simulink model "stereo_ibvs_core_backup_20260724_173834"  (R2025b)
settings: Solver=FixedStepDiscrete  StartTime=0.0  StopTime=10  FixedStep=cfg.Ts  RelTol=1e-3
InitFcn:
  | modelPath = get_param(bdroot,'FileName');
  |                                                                                       simulinkPath = fileparts(fileparts(modelPath));
  |                                                                                       configPath = fullfile(simulinkPath,'config','stereo_ibvs_config.m');
  |                                                                                       if ~isfile(configPath), error('StereoIBVS:ConfigNotFound','找不到配置文件：%s',configPath); end
  |                                                                                       run(configPath);
undefined symbols (not defined in the file): cfg
(part 3 of 4)

== matlab function stereo_ibvs_core_backup_20260724_173834/04_FR3_Camera_Kinematics/FR3 Camera Kinematics ==
  data: q input; pWCL output; cfg_T_W_B input; cfg_fr3OriginXYZ input; cfg_fr3OriginRPY input; cfg_fr3Axis input; cfg_fr3Joint8OriginXYZ input; cfg_fr3Joint8OriginRPY input; cfg_T_link8_CL input; cfg_T_CL_CR input; cfg_numericalEpsilon input; RWCL output; pWCR output; RWCR output; JL output; JR output; rankJL output; rcondJL output; rotationOrthogonalityError output; baselineLength output; baselineError output; stereoRotationError output; pWLink8 output; RWLink8 output; kinematicsValid output
function [ ...
    pWCL, ...
    RWCL, ...
    pWCR, ...
    RWCR, ...
    JL, ...
    JR, ...
    rankJL, ...
    rcondJL, ...
    rotationOrthogonalityError, ...
    baselineLength, ...
    baselineError, ...
    stereoRotationError, ...
    pWLink8, ...
    RWLink8, ...
    kinematicsValid] = fcn( ...
    q, ...
    cfg_T_W_B, ...
    cfg_fr3OriginXYZ, ...
    cfg_fr3OriginRPY, ...
    cfg_fr3Axis, ...
    cfg_fr3Joint8OriginXYZ, ...
    cfg_fr3Joint8OriginRPY, ...
    cfg_T_link8_CL, ...
    cfg_T_CL_CR, ...
    cfg_numericalEpsilon)
%#codegen
% V2 FR3双目相机运动学与诊断。

% 固定尺寸输出
pWCL = zeros(3,1);
RWCL = eye(3);
pWCR = zeros(3,1);
RWCR = eye(3);
JL = zeros(6,7);
JR = zeros(6,7);
rankJL = 0;
rcondJL = 0;
rotationOrthogonalityError = 0;
baselineLength = 0;
baselineError = 0;
stereoRotationError = 0;
pWLink8 = zeros(3,1);
RWLink8 = eye(3);
kinematicsValid = false;

% 输入整理和检查
qSafe = reshape(q,7,1);

inputValid = ...
    all(isfinite(qSafe)) && ...
    all(isfinite(cfg_T_W_B(:))) && ...
    all(isfinite(cfg_fr3OriginXYZ(:))) && ...
    all(isfinite(cfg_fr3OriginRPY(:))) && ...
    all(isfinite(cfg_fr3Axis(:))) && ...
    all(isfinite(cfg_fr3Joint8OriginXYZ(:))) && ...
    all(isfinite(cfg_fr3Joint8OriginRPY(:))) && ...
    all(isfinite(cfg_T_link8_CL(:))) && ...
    all(isfinite(cfg_T_CL_CR(:))) && ...
    isfinite(cfg_numericalEpsilon) && ...
    cfg_numericalEpsilon > 0;

if ~inputValid
    return;
end

% FR3正运动学
T = reshape(cfg_T_W_B,4,4);
jointOriginsW = zeros(3,7);
jointAxesW = zeros(3,7);

for jointIndex = 1:7
    T = T * makeTransform( ...
        cfg_fr3OriginXYZ(:,jointIndex), ...
        cfg_fr3OriginRPY(:,jointIndex));

    jointOriginsW(:,jointIndex) = T(1:3,4);

    axisLocal = cfg_fr3Axis(:,jointIndex);
    axisNorm = norm(axisLocal);

    if ~isfinite(axisNorm) || ...
            axisNorm <= cfg_numericalEpsilon
        return;
    end

    jointAxesW(:,jointIndex) = ...
        T(1:3,1:3) * axisLocal;

    T = T * axisRotation(axisLocal,qSafe(jointIndex));
end

% link8固定变换
T_W_link8 = T * makeTransform( ...
    cfg_fr3Joint8OriginXYZ, ...
    cfg_fr3Joint8OriginRPY);

pWLink8 = T_W_link8(1:3,4);
RWLink8 = T_W_link8(1:3,1:3);

% 左右相机位姿
T_W_CL = T_W_link8 * reshape(cfg_T_link8_CL,4,4);
T_W_CR = T_W_CL * reshape(cfg_T_CL_CR,4,4);

pWCL = T_W_CL(1:3,4);
RWCL = T_W_CL(1:3,1:3);
pWCR = T_W_CR(1:3,4);
RWCR = T_W_CR(1:3,1:3);

% 左相机光心的世界坐标Jacobian
JWLeft = zeros(6,7);

for jointIndex = 1:7
    JWLeft(1:3,jointIndex) = cross( ...
        jointAxesW(:,jointIndex), ...
        pWCL-jointOriginsW(:,jointIndex));

    JWLeft(4:6,jointIndex) = ...
        jointAxesW(:,jointIndex);
end

% 转换到左相机坐标系
R_CL_W = RWCL';

JL = [ ...
    R_CL_W, zeros(3,3)
    zeros(3,3), R_CL_W
    ] * JWLeft;

% 从左相机Jacobian转换到右相机坐标系
R_CL_CR = cfg_T_CL_CR(1:3,1:3);
p_CL_CR = cfg_T_CL_CR(1:3,4);

JR = [ ...
    R_CL_CR', -R_CL_CR'*skew3(p_CL_CR)
    zeros(3,3), R_CL_CR'
    ] * JL;

% 有限值检查
finiteResult = ...
    all(isfinite(pWCL)) && ...
    all(isfinite(RWCL(:))) && ...
    all(isfinite(pWCR)) && ...
    all(isfinite(RWCR(:))) && ...
    all(isfinite(JL(:))) && ...
    all(isfinite(JR(:))) && ...
    all(isfinite(pWLink8)) && ...
    all(isfinite(RWLink8(:)));

if ~finiteResult
    pWCL = zeros(3,1);
    RWCL = eye(3);
    pWCR = zeros(3,1);
    RWCR = eye(3);
    JL = zeros(6,7);
    JR = zeros(6,7);
    pWLink8 = zeros(3,1);
    RWLink8 = eye(3);
    return;
end

% V2运动学诊断
rankJL = rank(JL);
rcondJL = rcond(JL*JL');

rotationOrthogonalityError = max([ ...
    norm(RWCL'*RWCL-eye(3),'fro'), ...
    norm(RWCR'*RWCR-eye(3),'fro'), ...
    norm(RWLink8'*RWLink8-eye(3),'fro')]);

baselineLength = norm(pWCR-pWCL);
baselineError = abs( ...
    baselineLength-norm(p_CL_CR));

stereoRotationError = norm( ...
    RWCR-RWCL*R_CL_CR, ...
    'fro');

% 最终有效性判断
rotationTolerance = max( ...
    1e-6, ...
    100*cfg_numericalEpsilon);

diagnosticsFinite = ...
    isfinite(rankJL) && ...
    isfinite(rcondJL) && ...
    isfinite(rotationOrthogonalityError) && ...
    isfinite(baselineLength) && ...
    isfinite(baselineError) && ...
    isfinite(stereoRotationError);

rotationValid = ...
    rotationOrthogonalityError <= rotationTolerance && ...
    abs(det(RWCL)-1) <= rotationTolerance && ...
    abs(det(RWCR)-1) <= rotationTolerance && ...
    abs(det(RWLink8)-1) <= rotationTolerance;

kinematicsValid = ...
    diagnosticsFinite && ...
    rotationValid;

if ~kinematicsValid
    return;
end
end


function T = makeTransform(xyz,rpy)
T = eye(4);
T(1:3,1:3) = ...
    rotz3(rpy(3)) * ...
    roty3(rpy(2)) * ...
    rotx3(rpy(1));
T(1:3,4) = xyz;
end


function T = axisRotation(axis,q)
axisNorm = norm(axis);
unitAxis = axis / axisNorm;
K = skew3(unitAxis);
R = eye(3) + ...
    sin(q)*K + ...
    (1-cos(q))*(K*K);
T = eye(4);
T(1:3,1:3) = R;
end


function R = rotx3(angle)
c = cos(angle);
s = sin(angle);
R = [ ...
    1, 0, 0
    0, c, -s
    0, s, c
    ];
end


function R = roty3(angle)
c = cos(angle);
s = sin(angle);
R = [ ...
    c, 0, s
    0, 1, 0
    -s, 0, c
    ];
end


function R = rotz3(angle)
c = cos(angle);
s = sin(angle);
R = [ ...
    c, -s, 0
    s, c, 0
    0, 0, 1
    ];
end


function S = skew3(vector)
S = [ ...
    0, -vector(3), vector(2)
    vector(3), 0, -vector(1)
    -vector(2), vector(1), 0
    ];
end

== matlab function stereo_ibvs_core_backup_20260724_173834/05_Target_EKF/V2 Target EKF ==
  data: zMeasured input; pHatW output; measurementEnable input; visionMeasurementNewSafe input; pWCL input; RWCL input; fxMeasuredPx input; fyMeasuredPx input; resetSafe input; cfg_ekfX0 input; cfg_ekfP0 input; cfg_Ts input; cfg_sigmaJerk input; cfg_visibilityZMin input; cfg_numericalEpsilon input; cfg_rhoMin input; cfg_rhoMax input; cfg_pixelNoiseStd input; cfg_baseline input; cfg_ekfCovarianceJitter input; cfg_ekfSConditionMin input; cfg_ekfInitializationMode input; cfg_ekfRequireNewMeasurement input; vHatW output; aHatW output; pHatLeft output; vHatLeft output; rhoHatRaw output; rhoHatSafe output; innovation output; rhoInnovation output; innovationNorm output; traceP output; ekfPredictionValid output; ekfMeasurementUpdated output; ekfStateFinite output; minEigenvalueP output; symmetryErrorP output
function [ ...
    pHatW, ...
    vHatW, ...
    aHatW, ...
    pHatLeft, ...
    vHatLeft, ...
    rhoHatRaw, ...
    rhoHatSafe, ...
    innovation, ...
    rhoInnovation, ...
    innovationNorm, ...
    traceP, ...
    ekfPredictionValid, ...
    ekfMeasurementUpdated, ...
    ekfStateFinite, ...
    minEigenvalueP, ...
    symmetryErrorP] = fcn( ...
    zMeasured, ...
    measurementEnable, ...
    visionMeasurementNewSafe, ...
    pWCL, ...
    RWCL, ...
    fxMeasuredPx, ...
    fyMeasuredPx, ...
    resetSafe, ...
    cfg_ekfX0, ...
    cfg_ekfP0, ...
    cfg_Ts, ...
    cfg_sigmaJerk, ...
    cfg_visibilityZMin, ...
    cfg_numericalEpsilon, ...
    cfg_rhoMin, ...
    cfg_rhoMax, ...
    cfg_pixelNoiseStd, ...
    cfg_baseline, ...
    cfg_ekfCovarianceJitter, ...
    cfg_ekfSConditionMin, ...
    cfg_ekfInitializationMode, ...
    cfg_ekfRequireNewMeasurement)
%#codegen
% V2九状态世界坐标恒加速度EKF。
% 首次有效双目测量可直接初始化目标世界坐标位置。

% 固定尺寸输出
pHatW = zeros(3,1);
vHatW = zeros(3,1);
aHatW = zeros(3,1);
pHatLeft = zeros(3,1);
vHatLeft = zeros(3,1);
rhoHatRaw = 0;
rhoHatSafe = 0;
innovation = zeros(3,1);
rhoInnovation = 0;
innovationNorm = 0;
traceP = 0;
ekfPredictionValid = 0;
ekfMeasurementUpdated = 0;
ekfStateFinite = 0;
minEigenvalueP = 0;
symmetryErrorP = 0;

% 输入整理
z = reshape(zMeasured,3,1);
pCameraW = reshape(pWCL,3,1);
rotationCameraToWorld = reshape(RWCL,3,3);
fx = reshape(fxMeasuredPx,2,1);
fy = reshape(fyMeasuredPx,2,1);
ekfX0 = reshape(cfg_ekfX0,9,1);
ekfP0 = reshape(cfg_ekfP0,9,9);

% 持久状态
persistent x P initialized

if isempty(x)
    x = zeros(9,1);
    P = eye(9);
    initialized = false;
end

% 配置和输入有效性
configurationValid = ...
    all(isfinite(ekfX0)) && ...
    all(isfinite(ekfP0(:))) && ...
    isfinite(cfg_Ts) && cfg_Ts > 0 && ...
    isfinite(cfg_sigmaJerk) && cfg_sigmaJerk >= 0 && ...
    isfinite(cfg_visibilityZMin) && cfg_visibilityZMin > 0 && ...
    isfinite(cfg_numericalEpsilon) && cfg_numericalEpsilon > 0 && ...
    isfinite(cfg_rhoMin) && ...
    isfinite(cfg_rhoMax) && ...
    cfg_rhoMax > cfg_rhoMin && ...
    isfinite(cfg_pixelNoiseStd) && cfg_pixelNoiseStd >= 0 && ...
    isfinite(cfg_baseline) && ...
    cfg_baseline > cfg_numericalEpsilon && ...
    isfinite(cfg_ekfCovarianceJitter) && ...
    cfg_ekfCovarianceJitter >= 0 && ...
    isfinite(cfg_ekfSConditionMin) && ...
    cfg_ekfSConditionMin >= 0 && ...
    isfinite(cfg_ekfInitializationMode) && ...
    isfinite(cfg_ekfRequireNewMeasurement);

kinematicInputFinite = ...
    all(isfinite(pCameraW)) && ...
    all(isfinite(rotationCameraToWorld(:)));

focalPixelsValid = ...
    all(isfinite(fx)) && ...
    all(isfinite(fy)) && ...
    all(fx > cfg_numericalEpsilon) && ...
    all(fy > cfg_numericalEpsilon);

measurementEnableValid = ...
    isfinite(measurementEnable) && ...
    measurementEnable > 0.5;

visionNewValid = ...
    isfinite(visionMeasurementNewSafe) && ...
    visionMeasurementNewSafe > 0.5;

newMeasurementAccepted = ...
    cfg_ekfRequireNewMeasurement <= 0.5 || ...
    visionNewValid;

measurementFinite = all(isfinite(z));
measurementRhoValid = ...
    measurementFinite && ...
    z(3) >= cfg_rhoMin && ...
    z(3) <= cfg_rhoMax;

measurementAvailable = ...
    configurationValid && ...
    measurementEnableValid && ...
    newMeasurementAccepted && ...
    kinematicInputFinite && ...
    focalPixelsValid && ...
    measurementRhoValid;

resetRequested = ...
    isfinite(resetSafe) && ...
    resetSafe > 0.5;

if ~configurationValid
    initialized = false;
    return;
end

if resetRequested
    x = ekfX0;
    P = ekfP0;
    initialized = false;
    return;
end

% 固定初值模式兼容
fixedInitializationMode = ...
    cfg_ekfInitializationMode <= 0.5;

if ~initialized && fixedInitializationMode
    x = ekfX0;
    P = ekfP0;
    initialized = true;
end

% 首次有效双目测量初始化
justInitialized = false;

if ~initialized && measurementAvailable
    rhoInitial = z(3);
    depthInitial = 1/rhoInitial;

    pInitialLeft = [ ...
        z(1)*depthInitial
        z(2)*depthInitial
        depthInitial
    ];

    pInitialW = ...
        pCameraW + ...
        rotationCameraToWorld*pInitialLeft;

    initializationFinite = ...
        all(isfinite(pInitialLeft)) && ...
        all(isfinite(pInitialW)) && ...
        depthInitial > cfg_visibilityZMin;

    if initializationFinite
        x = [ ...
            pInitialW
            zeros(3,1)
            zeros(3,1)
        ];
        P = ekfP0;
        initialized = true;
        justInitialized = true;
        ekfMeasurementUpdated = 1;
    end
end

% 尚未初始化时保持安全无效输出
if ~initialized
    traceP = trace(0.5*(P+P'));
    return;
end

% 初始化当周期不重复执行预测和测量更新
if justInitialized
    pHatW = x(1:3);
    vHatW = x(4:6);
    aHatW = x(7:9);
    pHatLeft = ...
        rotationCameraToWorld' * ...
        (pHatW-pCameraW);
    vHatLeft = rotationCameraToWorld'*vHatW;

    ekfStateFinite = double( ...
        all(isfinite(x)) && ...
        all(isfinite(P(:))) && ...
        all(isfinite(pHatLeft)) && ...
        all(isfinite(vHatLeft)));

    if ekfStateFinite > 0.5 && ...
            pHatLeft(3) > cfg_visibilityZMin
        rhoHatRaw = 1/pHatLeft(3);
        rhoHatSafe = min( ...
            max(rhoHatRaw,cfg_rhoMin), ...
            cfg_rhoMax);
        ekfPredictionValid = 1;
    end

    Psym = 0.5*(P+P');
    traceP = trace(Psym);
    symmetryErrorP = norm(P-P','fro');
    eigenvaluesP = eig(Psym);
    minEigenvalueP = min(real(eigenvaluesP));
    return;
end

% 恒加速度状态模型
I3 = eye(3);
Z3 = zeros(3,3);
I9 = eye(9);
Ts = cfg_Ts;

F = [ ...
    I3, Ts*I3, 0.5*Ts*Ts*I3
    Z3, I3,    Ts*I3
    Z3, Z3,    I3
];

sigmaJerkSquared = cfg_sigmaJerk*cfg_sigmaJerk;

Q = sigmaJerkSquared * [ ...
    (Ts^5/20)*I3, (Ts^4/8)*I3, (Ts^3/6)*I3
    (Ts^4/8)*I3,  (Ts^3/3)*I3, (Ts^2/2)*I3
    (Ts^3/6)*I3,  (Ts^2/2)*I3, Ts*I3
];

% 预测
xPred = F*x;
PPred = F*P*F' + Q;
PPred = 0.5*(PPred+PPred');

pPredW = xPred(1:3);
pPredLeft = ...
    rotationCameraToWorld' * ...
    (pPredW-pCameraW);

predictionFinite = ...
    kinematicInputFinite && ...
    all(isfinite(xPred)) && ...
    all(isfinite(PPred(:))) && ...
    all(isfinite(pPredLeft));

ekfPredictionValid = double( ...
    predictionFinite && ...
    pPredLeft(3) > cfg_visibilityZMin);

% 默认采用预测结果
x = xPred;
P = PPred;

% 仅在新视觉消息到来时执行测量更新
measurementOK = ...
    measurementAvailable && ...
    ekfPredictionValid > 0.5;

if measurementOK
    Z = pPredLeft(3);
    rhoPred = 1/Z;
    xLeftPred = pPredLeft(1)/Z;
    yLeftPred = pPredLeft(2)/Z;

    h = [xLeftPred; yLeftPred; rhoPred];

    HLeft = [ ...
        rhoPred, 0,       -xLeftPred*rhoPred
        0,       rhoPred, -yLeftPred*rhoPred
        0,       0,       -rhoPred*rhoPred
    ];

    HWorld = HLeft*rotationCameraToWorld';
    H = [HWorld, zeros(3,3), zeros(3,3)];

    if all(isfinite(h)) && all(isfinite(H(:)))
        innovation = z-h;
        rhoInnovation = innovation(3);

        pixelVariance = ...
            cfg_pixelNoiseStd*cfg_pixelNoiseStd;
        fxLeft = max(fx(1),cfg_numericalEpsilon);
        fxRight = max(fx(2),cfg_numericalEpsilon);
        fyLeft = max(fy(1),cfg_numericalEpsilon);
        baseline = max(cfg_baseline,cfg_numericalEpsilon);

        varXLeft = pixelVariance/(fxLeft*fxLeft);
        varYLeft = pixelVariance/(fyLeft*fyLeft);
        covXLeftRho = ...
            pixelVariance/(baseline*fxLeft*fxLeft);
        varRho = pixelVariance/(baseline*baseline) * ...
            (1/(fxLeft*fxLeft)+1/(fxRight*fxRight));

        R = [ ...
            varXLeft,    0,        covXLeftRho
            0,           varYLeft, 0
            covXLeftRho, 0,        varRho
        ];

        R = R + cfg_ekfCovarianceJitter*eye(3);
        S = H*PPred*H' + R;

        innovationCovarianceValid = ...
            all(isfinite(S(:))) && ...
            rcond(S) > cfg_ekfSConditionMin;

        if innovationCovarianceValid
            K = (PPred*H')/S;
            xUpdated = xPred+K*innovation;
            A = I9-K*H;
            PUpdated = A*PPred*A'+K*R*K';
            PUpdated = 0.5*(PUpdated+PUpdated');

            if cfg_ekfCovarianceJitter > 0
                PUpdated = PUpdated + ...
                    cfg_ekfCovarianceJitter*I9;
            end

            updateFinite = ...
                all(isfinite(xUpdated)) && ...
                all(isfinite(PUpdated(:)));

            if updateFinite
                x = xUpdated;
                P = PUpdated;
                ekfMeasurementUpdated = 1;
            end
        end
    end
end

% 状态输出
pHatW = x(1:3);
vHatW = x(4:6);
aHatW = x(7:9);
pHatLeft = ...
    rotationCameraToWorld' * ...
    (pHatW-pCameraW);
vHatLeft = rotationCameraToWorld'*vHatW;

ekfStateFinite = double( ...
    all(isfinite(x)) && ...
    all(isfinite(P(:))) && ...
    all(isfinite(pHatLeft)) && ...
    all(isfinite(vHatLeft)));

if ekfStateFinite > 0.5 && ...
        pHatLeft(3) > cfg_visibilityZMin
    rhoHatRaw = 1/pHatLeft(3);
    rhoHatSafe = min( ...
        max(rhoHatRaw,cfg_rhoMin), ...
        cfg_rhoMax);
else
    rhoHatRaw = 0;
    rhoHatSafe = 0;
    ekfPredictionValid = 0;
end

innovationNorm = sqrt(innovation'*innovation);
Psym = 0.5*(P+P');
symmetryErrorP = norm(P-P','fro');
traceP = trace(Psym);
eigenvaluesP = eig(Psym);
minEigenvalueP = min(real(eigenvaluesP));

% 非有限状态自动复位并重新等待初始化
diagnosticsValid = ...
    ekfStateFinite > 0.5 && ...
    isfinite(traceP) && ...
    isfinite(minEigenvalueP) && ...
    isfinite(symmetryErrorP);

if ~diagnosticsValid
    x = ekfX0;
    P = ekfP0;
    initialized = false;

    pHatW = zeros(3,1);
    vHatW = zeros(3,1);
    aHatW = zeros(3,1);
    pHatLeft = zeros(3,1);
    vHatLeft = zeros(3,1);
    rhoHatRaw = 0;
    rhoHatSafe = 0;
    innovation = zeros(3,1);
    rhoInnovation = 0;
    innovationNorm = 0;
    traceP = trace(ekfP0);
    minEigenvalueP = 0;
    symmetryErrorP = 0;
    ekfPredictionValid = 0;
    ekfMeasurementUpdated = 0;
    ekfStateFinite = 0;
end
end

== matlab function stereo_ibvs_core_backup_20260724_173834/06_Estimated_Rho_Dynamics/Estimate Rho Dynamics ==
  data: normalizedFeatureMeasured input; rhoDotHat output; rhoHatSafe input; vHatCL input; vHatCR input; JL input; JR input; qDotMeasured input; motionFeedbackValid input; cfg_numericalEpsilon input; rhoDynamicsValid output
function [rhoDotHat, rhoDynamicsValid] = fcn( ...
    normalizedFeatureMeasured, ...
    rhoHatSafe, ...
    vHatCL, ...
    vHatCR, ...
    JL, ...
    JR, ...
    qDotMeasured, ...
    motionFeedbackValid, ...
    cfg_numericalEpsilon)
%#codegen
% 本函数使用实测关节速度估计左右相机运动引起的逆深度变化率。
%
% 输入尺寸：
% normalizedFeatureMeasured : 4×1 [xL;yL;xR;yR]
% rhoHatSafe                : 1×1
% vHatCL                    : 3×1
% vHatCR                    : 3×1
% JL                        : 6×7
% JR                        : 6×7
% qDotMeasured              : 7×1，来自JointState.velocity
% motionFeedbackValid       : 1×1
%
% 输出：
% rhoDotHat                 : 2×1
% rhoDynamicsValid          : 1×1

%% 固定尺寸输出
rhoDotHat = zeros(2,1);
rhoDynamicsValid = false;

features = reshape(normalizedFeatureMeasured,4,1);
velocityCL = reshape(vHatCL,3,1);
velocityCR = reshape(vHatCR,3,1);
qDotFeedback = reshape(qDotMeasured,7,1);

%% 输入有效性
inputValid = ...
    all(isfinite(features)) && ...
    isfinite(rhoHatSafe) && ...
    all(isfinite(velocityCL)) && ...
    all(isfinite(velocityCR)) && ...
    all(isfinite(JL(:))) && ...
    all(isfinite(JR(:))) && ...
    all(isfinite(qDotFeedback)) && ...
    isfinite(motionFeedbackValid) && ...
    motionFeedbackValid > 0.5 && ...
    isfinite(cfg_numericalEpsilon) && ...
    cfg_numericalEpsilon > 0 && ...
    rhoHatSafe > cfg_numericalEpsilon;

if ~inputValid
    return;
end

rho = max(rhoHatSafe, cfg_numericalEpsilon);

%% 左相机
xL = features(1);
yL = features(2);

LrhoL = [
    0, 0, rho*rho, ...
    rho*yL, -rho*xL, 0
];

Hrho = [0, 0, -rho*rho];

cameraVelocityLeft = JL * qDotFeedback;

rhoDotHat(1) = ...
    LrhoL * cameraVelocityLeft + ...
    Hrho * velocityCL;

%% 右相机
xR = features(3);
yR = features(4);

LrhoR = [
    0, 0, rho*rho, ...
    rho*yR, -rho*xR, 0
];

cameraVelocityRight = JR * qDotFeedback;

rhoDotHat(2) = ...
    LrhoR * cameraVelocityRight + ...
    Hrho * velocityCR;

%% 最终数值保护
if all(isfinite(rhoDotHat))
    rhoDynamicsValid = true;
else
    rhoDotHat = zeros(2,1);
    rhoDynamicsValid = false;
end
end

== matlab function stereo_ibvs_core_backup_20260724_173834/07_Arm_Priority_Controller/Final Arm Priority Controller ==
  data: q input; qDotCmd output; cLMeasured input; rhoHatL input; vHatLeft input; JL input; cLd input; rhoD input; validLeft input; ekfPredictionValid input; centerEnable input; depthEnable input; armEnable input; depthTaskWeight input; cfg_numericalEpsilon input; cfg_robustEnable input; cfg_betaC input; cfg_epsilonC input; cfg_Kc input; cfg_lambdaC input; cfg_betaRho input; cfg_epsilonRho input; cfg_kRho input; cfg_lambdaRho input; cfg_nullspaceEnable input; cfg_kNull input; cfg_qMid input; cfg_leftOnlyCenterControlEnable input; centerError output; depthError output; rcondJc output; rcondArho output; qDotCenter output; qDotDepthRaw output; qDotDepthWeighted output; qDotNullUsed output
function [qDotCmd,centerError,depthError,rcondJc,rcondArho,qDotCenter,qDotDepthRaw,qDotDepthWeighted,qDotNullUsed] = ...
    fcn(q,cLMeasured,rhoHatL,vHatLeft,JL,cLd,rhoD,validLeft,ekfPredictionValid,centerEnable,depthEnable,armEnable,depthTaskWeight, ...
    cfg_numericalEpsilon,cfg_robustEnable,cfg_betaC,cfg_epsilonC,cfg_Kc,cfg_lambdaC,cfg_betaRho,cfg_epsilonRho,cfg_kRho,cfg_lambdaRho,cfg_nullspaceEnable,cfg_kNull,cfg_qMid,cfg_leftOnlyCenterControlEnable)
%#codegen
% 代码作用：
% 左相机归一化中心为主任务，逆深度为次任务。
% 支持目标速度前馈、鲁棒项、阻尼伪逆和关节中位零空间任务。

qDotCmd = zeros(7,1);
centerError = zeros(2,1);
depthError = 0;
rcondJc = 0;
rcondArho = 0;
qDotCenter = zeros(7,1);
qDotDepthRaw = zeros(7,1);
qDotDepthWeighted = zeros(7,1);
qDotNullUsed = zeros(7,1);

x = cLMeasured(1);
y = cLMeasured(2);
rho = rhoD;
vFeed = zeros(3,1);

if ekfPredictionValid > 0.5 && ...
        isfinite(rhoHatL) && rhoHatL > 0 && ...
        all(isfinite(vHatLeft))
    rho = max(rhoHatL,cfg_numericalEpsilon);
    vFeed = vHatLeft;
end

centerError = [x;y] - cLd;
depthError = rho - rhoD;

Lc = [
    -rho, 0, x*rho, x*y, -(1+x*x), y
    0, -rho, y*rho, 1+y*y, -x*y, -x
];

Hc = rho*[1 0 -x;0 1 -y];
bhatC = Hc*vFeed;
Jc = Lc*JL;

rc = zeros(2,1);
if cfg_robustEnable > 0.5
    rc = cfg_betaC*centerError / ...
        (sqrt(centerError'*centerError)+cfg_epsilonC);
end

nuC = -cfg_Kc*centerError - bhatC - rc;
Gc = Jc*Jc' + cfg_lambdaC^2*eye(2);
JcSharp = Jc'/Gc;
qC = JcSharp*nuC;
Nc = eye(7)-JcSharp*Jc;
rcondJc = det(Gc) / ...
    (trace(Gc)*trace(Gc)+cfg_numericalEpsilon);
qDotCenter = qC;

Lrho = [0 0 rho*rho rho*y -rho*x 0];
Hrho = [0 0 -rho*rho];
Jrho = Lrho*JL;
bhatRho = Hrho*vFeed;

rr = 0;
if cfg_robustEnable > 0.5
    rr = cfg_betaRho*depthError / ...
        (abs(depthError)+cfg_epsilonRho);
end

nuRho = -cfg_kRho*depthError-bhatRho-rr;
A = Jrho*Nc;
denom = A*A'+cfg_lambdaRho^2;
rcondArho = denom/(1+denom);

w = min(max(depthTaskWeight,0),1) * ...
    double(ekfPredictionValid > 0.5);
qDotDepthRaw = Nc*A'*((nuRho-Jrho*qC)/denom);
qDotDepthWeighted = w*qDotDepthRaw;

qDot0 = zeros(7,1);
if cfg_nullspaceEnable > 0.5
    qDot0 = -cfg_kNull*(q-cfg_qMid);
end

ArhoDagger = A'/denom;
NcRho = Nc*(eye(7)-ArhoDagger*A);
Nnull = (1-w)*Nc+w*NcRho;
qDotNullUsed = Nnull*qDot0;

if centerEnable > 0.5
    qDotCmd = qDotCenter+qDotNullUsed;
end

if centerEnable > 0.5 && depthEnable > 0.5
    qDotCmd = qDotCenter+qDotDepthWeighted+qDotNullUsed;
end

if centerEnable <= 0.5 && depthEnable > 0.5
    d = Jrho*Jrho'+cfg_lambdaRho^2;
    qDotDepthRaw = Jrho'*(nuRho/d);
    qDotDepthWeighted = w*qDotDepthRaw;
    qDotCenter = zeros(7,1);
    qDotNullUsed = zeros(7,1);
    qDotCmd = qDotDepthWeighted;
end

centerAllowed = validLeft > 0.5 && ...
    cfg_leftOnlyCenterControlEnable > 0.5;

if ~centerAllowed || armEnable <= 0.5
    qDotCmd = zeros(7,1);
    qDotCenter = zeros(7,1);
    qDotDepthWeighted = zeros(7,1);
    qDotNullUsed = zeros(7,1);
end

if any(~isfinite(qDotCmd))
    qDotCmd = zeros(7,1);
end
end

== matlab function stereo_ibvs_core_backup_20260724_173834/08_Zoom_Controller/08A Right Visibility Guard/Right Visibility Guard ==
  data: xLeftMeasured input; uRightPredicted output; rhoHatSafe input; focalLengthMeasuredMm input; focalLengthDataValid input; cameraModelValid input; validLeft input; validRight input; ekfPredictionValid input; rightReacquireActive input; resetSafe input; scaleDesired input; numericalEpsilon input; baseline input; outputPixelPitchXmm input; cxR input; focalLengthHardwareMaxMm input; visibilityEpsilon input; imageWidthPx input; rightVisibilityMarginPx input; focalLengthWorkingMaxMm input; focalLengthWorkingMinMm input; targetCharacteristicSize input; rightVisibilityHysteresisPx input; rightVisibilityMarginActualPx output; fRightMaxVisibleMm output; fRightMaxEffectiveMm output; rightScaleDesiredEffective output; rightVisibilityActive output; rightVisibilityInfeasible output; scaleDesiredEffective output; rightScaleDesiredNominal output; fRightMeasuredMm output
function [ ...
    uRightPredicted, ...
    rightVisibilityMarginActualPx, ...
    fRightMaxVisibleMm, ...
    fRightMaxEffectiveMm, ...
    rightScaleDesiredEffective, ...
    rightVisibilityActive, ...
    rightVisibilityInfeasible, ...
    scaleDesiredEffective, ...
    rightScaleDesiredNominal, ...
    fRightMeasuredMm] = fcn( ...
    xLeftMeasured, ...
    rhoHatSafe, ...
    focalLengthMeasuredMm, ...
    focalLengthDataValid, ...
    cameraModelValid, ...
    validLeft, ...
    validRight, ...
    ekfPredictionValid, ...
    rightReacquireActive, ...
    resetSafe, ...
    scaleDesired, ...
    numericalEpsilon, ...
    baseline, ...
    outputPixelPitchXmm, ...
    cxR, ...
    focalLengthHardwareMaxMm, ...
    visibilityEpsilon, ...
    imageWidthPx, ...
    rightVisibilityMarginPx, ...
    focalLengthWorkingMaxMm, ...
    focalLengthWorkingMinMm, ...
    targetCharacteristicSize, ...
    rightVisibilityHysteresisPx)
%#codegen
% 右相机可见性保护。
% 所有配置参数均由外部 Constant 块输入。

persistent active

if isempty(active)
    active = 1;
end

if resetSafe > 0.5
    active = 1;
end

%% 默认安全输出
uRightPredicted = cxR;
rightVisibilityMarginActualPx = 0;

fRightMaxVisibleMm = 0;
fRightMaxEffectiveMm = ...
    focalLengthWorkingMinMm(2);

rightScaleDesiredNominal = ...
    scaleDesired(2);

rightScaleDesiredEffective = ...
    rightScaleDesiredNominal;

scaleDesiredEffective = ...
    scaleDesired;

rightVisibilityActive = 1;
rightVisibilityInfeasible = 1;

fRightMeasuredMm = 0;

%% 输入检查
inputFinite = ...
    isfinite(xLeftMeasured) && ...
    isfinite(rhoHatSafe) && ...
    all(isfinite(focalLengthMeasuredMm)) && ...
    all(isfinite(scaleDesired)) && ...
    isfinite(numericalEpsilon) && ...
    isfinite(baseline) && ...
    isfinite(outputPixelPitchXmm) && ...
    isfinite(cxR) && ...
    all(isfinite(focalLengthHardwareMaxMm)) && ...
    isfinite(visibilityEpsilon) && ...
    isfinite(imageWidthPx) && ...
    isfinite(rightVisibilityMarginPx) && ...
    all(isfinite(focalLengthWorkingMaxMm)) && ...
    all(isfinite(focalLengthWorkingMinMm)) && ...
    isfinite(targetCharacteristicSize) && ...
    isfinite(rightVisibilityHysteresisPx);

modelReady = ...
    focalLengthDataValid > 0.5 && ...
    cameraModelValid > 0.5 && ...
    outputPixelPitchXmm > numericalEpsilon;

if ~inputFinite || ~modelReady
    active = 1;
    return;
end

%% 右相机预测位置
fRightMeasuredMm = ...
    focalLengthMeasuredMm(2);

rho = max( ...
    rhoHatSafe, ...
    numericalEpsilon);

xRightPredicted = ...
    xLeftMeasured - ...
    baseline * rho;

fRightPx = ...
    focalLengthMeasuredMm(2) / ...
    outputPixelPitchXmm;

uRightPredicted = ...
    cxR + ...
    fRightPx * xRightPredicted;

rightVisibilityMarginActualPx = min( ...
    uRightPredicted, ...
    imageWidthPx - uRightPredicted);

%% 可见焦距上限
hardwareMaxPx = ...
    focalLengthHardwareMaxMm(2) / ...
    outputPixelPitchXmm;

if xRightPredicted < -visibilityEpsilon

    fMaxPx = ...
        (cxR - rightVisibilityMarginPx) / ...
        (-xRightPredicted);

elseif xRightPredicted > visibilityEpsilon

    fMaxPx = ...
        (imageWidthPx - ...
        rightVisibilityMarginPx - ...
        cxR) / ...
        xRightPredicted;

else
    fMaxPx = hardwareMaxPx;
end

fMaxPx = max(fMaxPx, 0);

fRightMaxVisibleMm = ...
    fMaxPx * outputPixelPitchXmm;

rawEffectiveMaxMm = min([
    focalLengthWorkingMaxMm(2)
    focalLengthHardwareMaxMm(2)
    fRightMaxVisibleMm
]);

rightVisibilityInfeasible = double( ...
    rawEffectiveMaxMm < ...
    focalLengthWorkingMinMm(2));

fRightMaxEffectiveMm = max( ...
    focalLengthWorkingMinMm(2), ...
    rawEffectiveMaxMm);

%% 调整右相机期望尺度
scaleRightMaxVisible = ...
    targetCharacteristicSize * ...
    fMaxPx * rho;

rightScaleDesiredEffective = min( ...
    rightScaleDesiredNominal, ...
    max(scaleRightMaxVisible, numericalEpsilon));

scaleDesiredEffective = [
    scaleDesired(1)
    rightScaleDesiredEffective
];

%% 滞回状态
enterGuard = ...
    validLeft <= 0.5 || ...
    validRight <= 0.5 || ...
    ekfPredictionValid <= 0.5 || ...
    rightReacquireActive > 0.5 || ...
    rightVisibilityInfeasible > 0.5 || ...
    uRightPredicted < rightVisibilityMarginPx || ...
    uRightPredicted > ...
        imageWidthPx - rightVisibilityMarginPx || ...
    focalLengthMeasuredMm(2) > ...
        fRightMaxEffectiveMm + numericalEpsilon;

exitGuard = ...
    validLeft > 0.5 && ...
    validRight > 0.5 && ...
    ekfPredictionValid > 0.5 && ...
    rightReacquireActive <= 0.5 && ...
    rightVisibilityInfeasible <= 0.5 && ...
    uRightPredicted >= ...
        rightVisibilityMarginPx + ...
        rightVisibilityHysteresisPx && ...
    uRightPredicted <= ...
        imageWidthPx - ...
        rightVisibilityMarginPx - ...
        rightVisibilityHysteresisPx && ...
    focalLengthMeasuredMm(2) <= ...
        fRightMaxEffectiveMm;

if enterGuard
    active = 1;
elseif exitGuard
    active = 0;
end

rightVisibilityActive = ...
    double(active > 0.5);

%% 输出保护
if any(~isfinite([
        uRightPredicted
        rightVisibilityMarginActualPx
        fRightMaxVisibleMm
        fRightMaxEffectiveMm
        rightScaleDesiredEffective
        scaleDesiredEffective
        fRightMeasuredMm]))

    active = 1;

    uRightPredicted = cxR;
    rightVisibilityMarginActualPx = 0;

    fRightMaxVisibleMm = 0;
    fRightMaxEffectiveMm = ...
        focalLengthWorkingMinMm(2);

    rightScaleDesiredEffective = ...
        numericalEpsilon;

    scaleDesiredEffective = [
        scaleDesired(1)
        rightScaleDesiredEffective
    ];

    rightVisibilityActive = 1;
    rightVisibilityInfeasible = 1;
    fRightMeasuredMm = 0;
end
end

== matlab function stereo_ibvs_core_backup_20260724_173834/08_Zoom_Controller/08B_Zoom_Controller_Mm/V2 Zoom Controller ==
  data: focalLengthMeasuredMm input; fDotMmCmd output; focalLengthFresh input; focalLengthDataValid input; cameraModelValid input; scaleMeasured input; rhoHatSafe input; rhoDotHat input; scaleDesiredEffective input; validLeft input; ekfPredictionValid input; focalAtWorkingLowerLimit input; focalAtWorkingUpperLimit input; fRightMaxEffectiveMm input; rightVisibilityActive input; rightReacquireActive input; numericalEpsilon input; focalLengthWorkingMaxMm input; robustEnable input; betaF input; epsilonF input; Kf input; targetCharacteristicSize input; outputPixelPitchXmm input; focalLengthWorkingMinMm input; rightReacquireZoomRateMmPerSec input; focalRateDesignMmPerSec input; Ts input; focalRateGuaranteedMmPerSec input; focalRateAbsoluteMaxMmPerSec input; zoomControlEnable input; fDotMmLimited output; scaleError output; gDotCmd output; focalCommandOutwardAtWorkingLimit output; focalFeasible output; focalRateUsageGuaranteedCmd output; focalRateUsageHardCmd output
function [ ...
    fDotMmCmd, ...
    fDotMmLimited, ...
    scaleError, ...
    gDotCmd, ...
    focalCommandOutwardAtWorkingLimit, ...
    focalFeasible, ...
    focalRateUsageGuaranteedCmd, ...
    focalRateUsageHardCmd] = fcn( ...
    focalLengthMeasuredMm, ...
    focalLengthFresh, ...
    focalLengthDataValid, ...
    cameraModelValid, ...
    scaleMeasured, ...
    rhoHatSafe, ...
    rhoDotHat, ...
    scaleDesiredEffective, ...
    validLeft, ...
    ekfPredictionValid, ...
    focalAtWorkingLowerLimit, ...
    focalAtWorkingUpperLimit, ...
    fRightMaxEffectiveMm, ...
    rightVisibilityActive, ...
    rightReacquireActive, ...
    numericalEpsilon, ...
    focalLengthWorkingMaxMm, ...
    robustEnable, ...
    betaF, ...
    epsilonF, ...
    Kf, ...
    targetCharacteristicSize, ...
    outputPixelPitchXmm, ...
    focalLengthWorkingMinMm, ...
    rightReacquireZoomRateMmPerSec, ...
    focalRateDesignMmPerSec, ...
    Ts, ...
    focalRateGuaranteedMmPerSec, ...
    focalRateAbsoluteMaxMmPerSec, ...
    zoomControlEnable)
%#codegen
% V2 Zoom控制器。
% 焦距单位mm，速度命令单位mm/s。
% 所有配置参数均由外部 Constant 块输入。

%% 固定尺寸输出
fDotMmCmd = zeros(2,1);
fDotMmLimited = zeros(2,1);

scaleError = zeros(2,1);
gDotCmd = zeros(2,1);

focalCommandOutwardAtWorkingLimit = ...
    zeros(2,1);

focalFeasible = zeros(2,1);

focalRateUsageGuaranteedCmd = ...
    zeros(2,1);

focalRateUsageHardCmd = ...
    zeros(2,1);

%% 输入检查
inputFinite = ...
    all(isfinite(focalLengthMeasuredMm)) && ...
    all(isfinite(scaleMeasured)) && ...
    isfinite(rhoHatSafe) && ...
    all(isfinite(rhoDotHat)) && ...
    all(isfinite(scaleDesiredEffective)) && ...
    all(isfinite(focalAtWorkingLowerLimit)) && ...
    all(isfinite(focalAtWorkingUpperLimit)) && ...
    isfinite(fRightMaxEffectiveMm) && ...
    isfinite(numericalEpsilon) && ...
    all(isfinite(focalLengthWorkingMaxMm)) && ...
    isfinite(robustEnable) && ...
    all(isfinite(betaF)) && ...
    all(isfinite(epsilonF)) && ...
    all(isfinite(Kf(:))) && ...
    isfinite(targetCharacteristicSize) && ...
    isfinite(outputPixelPitchXmm) && ...
    all(isfinite(focalLengthWorkingMinMm)) && ...
    isfinite(rightReacquireZoomRateMmPerSec) && ...
    isfinite(focalRateDesignMmPerSec) && ...
    isfinite(Ts) && ...
    isfinite(focalRateGuaranteedMmPerSec) && ...
    isfinite(focalRateAbsoluteMaxMmPerSec) && ...
    isfinite(zoomControlEnable);

if ~inputFinite || ...
        numericalEpsilon <= 0 || ...
        outputPixelPitchXmm <= numericalEpsilon || ...
        Ts <= 0

    return;
end

rho = max(rhoHatSafe, numericalEpsilon);

upperEffectiveMm = [
    focalLengthWorkingMaxMm(1)
    fRightMaxEffectiveMm
];

%% V2控制律
for cameraIndex = 1:2

    scaleCurrent = max( ...
        scaleMeasured(cameraIndex), ...
        numericalEpsilon);

    scaleDesiredCurrent = max( ...
        scaleDesiredEffective(cameraIndex), ...
        numericalEpsilon);

    scaleError(cameraIndex) = ...
        log(scaleCurrent / scaleDesiredCurrent);

    depthRateEstimate = ...
        rhoDotHat(cameraIndex) / rho;

    robustTerm = 0;

    if robustEnable > 0.5
        robustTerm = ...
            betaF(cameraIndex) * ...
            scaleError(cameraIndex) / ...
            (abs(scaleError(cameraIndex)) + ...
            epsilonF(cameraIndex));
    end

    gDotCmd(cameraIndex) = ...
        -Kf(cameraIndex,cameraIndex) * ...
        scaleError(cameraIndex) - ...
        depthRateEstimate - ...
        robustTerm;

    fDotMmCmd(cameraIndex) = ...
        focalLengthMeasuredMm(cameraIndex) * ...
        gDotCmd(cameraIndex);

    focalRequiredMm = ...
        scaleDesiredEffective(cameraIndex) / ...
        (targetCharacteristicSize * rho) * ...
        outputPixelPitchXmm;

    focalFeasible(cameraIndex) = double( ...
        focalRequiredMm >= ...
            focalLengthWorkingMinMm(cameraIndex) && ...
        focalRequiredMm <= ...
            upperEffectiveMm(cameraIndex));
end

%% 焦距反馈超时或模型失效：Zoom立即停止
zoomInputValid = ...
    focalLengthFresh > 0.5 && ...
    focalLengthDataValid > 0.5 && ...
    cameraModelValid > 0.5;

if ~zoomInputValid || ...
        zoomControlEnable <= 0.5

    fDotMmCmd = zeros(2,1);
    fDotMmLimited = zeros(2,1);
    gDotCmd = zeros(2,1);
    return;
end

%% 右相机可见性保护
if rightVisibilityActive > 0.5 || ...
        rightReacquireActive > 0.5

    if focalLengthMeasuredMm(2) > ...
            fRightMaxEffectiveMm + numericalEpsilon

        fDotMmCmd(2) = ...
            -rightReacquireZoomRateMmPerSec;
    else
        fDotMmCmd(2) = ...
            min(fDotMmCmd(2), 0);
    end
end

%% 左相机或EKF无效：保留V2安全缩焦
if validLeft <= 0.5 || ...
        ekfPredictionValid <= 0.5

    fDotMmCmd = zeros(2,1);

    for cameraIndex = 1:2
        if focalLengthMeasuredMm(cameraIndex) > ...
                focalLengthWorkingMinMm(cameraIndex)

            fDotMmCmd(cameraIndex) = ...
                -rightReacquireZoomRateMmPerSec;
        end
    end
end

%% 工作范围方向诊断
for cameraIndex = 1:2

    focalCommandOutwardAtWorkingLimit(cameraIndex) = ...
        double( ...
        (focalAtWorkingLowerLimit(cameraIndex) > 0.5 && ...
        fDotMmCmd(cameraIndex) < 0) || ...
        (focalAtWorkingUpperLimit(cameraIndex) > 0.5 && ...
        fDotMmCmd(cameraIndex) > 0) || ...
        (focalLengthMeasuredMm(cameraIndex) >= ...
        upperEffectiveMm(cameraIndex) && ...
        fDotMmCmd(cameraIndex) > 0));
end

%% V2设计速度限制
fDotMmLimited = min( ...
    max( ...
        fDotMmCmd, ...
        -focalRateDesignMmPerSec), ...
    focalRateDesignMmPerSec);

%% 防止下一周期越过右相机可见焦距上限
nextRightFocalLengthMm = ...
    focalLengthMeasuredMm(2) + ...
    Ts * fDotMmLimited(2);

if focalLengthMeasuredMm(2) <= ...
        fRightMaxEffectiveMm && ...
        nextRightFocalLengthMm > ...
        fRightMaxEffectiveMm

    fDotMmLimited(2) = min( ...
        fDotMmLimited(2), ...
        (fRightMaxEffectiveMm - ...
        focalLengthMeasuredMm(2)) / Ts);
end

%% 速度使用率
if focalRateGuaranteedMmPerSec > numericalEpsilon
    focalRateUsageGuaranteedCmd = ...
        abs(fDotMmLimited) / ...
        focalRateGuaranteedMmPerSec;
end

if focalRateAbsoluteMaxMmPerSec > numericalEpsilon
    focalRateUsageHardCmd = ...
        abs(fDotMmLimited) / ...
        focalRateAbsoluteMaxMmPerSec;
end

%% 输出有限值保护
if any(~isfinite(fDotMmCmd)) || ...
        any(~isfinite(fDotMmLimited)) || ...
        any(~isfinite(scaleError)) || ...
        any(~isfinite(gDotCmd)) || ...
        any(~isfinite(focalFeasible)) || ...
        any(~isfinite(focalRateUsageGuaranteedCmd)) || ...
        any(~isfinite(focalRateUsageHardCmd))

    fDotMmCmd = zeros(2,1);
    fDotMmLimited = zeros(2,1);

    scaleError = zeros(2,1);
    gDotCmd = zeros(2,1);

    focalCommandOutwardAtWorkingLimit = ...
        zeros(2,1);

    focalFeasible = zeros(2,1);

    focalRateUsageGuaranteedCmd = ...
        zeros(2,1);

    focalRateUsageHardCmd = ...
        zeros(2,1);
end
end

== matlab function stereo_ibvs_core_backup_20260724_173834/08_Zoom_Controller/08C_Zoom_Priority_Supervisor/V2 Zoom Priority Supervisor ==
  data: scaleError input; depthTaskWeight output; depthErrorDelayed input; focalLengthMeasuredMm input; focalLengthFresh input; focalLengthDataValid input; cameraModelValid input; focalAtWorkingLowerLimit input; focalAtWorkingUpperLimit input; focalHeadroomMm input; focalFeasible input; validLeft input; validStereoQualified input; ekfPredictionValid input; resetSafe input; focalCommandOutwardAtWorkingLimit input; focalRateUsageGuaranteedCmd input; focalRateUsageHardCmd input; rightReacquireActive input; Ts input; zoomPriorityEnable input; armDepthRampTime input; scaleErrorEnterThreshold input; scaleErrorExitThreshold input; scaleSettledHoldTime input; disturbanceConfirmTime input; zoomOnlyMaxTime input; schedulerMode output; zoomPriorityActive output; zoomPriorityTimer output; scaleSettledTimer output; armRecoveryReason output; newDisturbanceDetected output
function [ ...
    depthTaskWeight, ...
    schedulerMode, ...
    zoomPriorityActive, ...
    zoomPriorityTimer, ...
    scaleSettledTimer, ...
    armRecoveryReason, ...
    newDisturbanceDetected] = fcn( ...
    scaleError, ...
    depthErrorDelayed, ...
    focalLengthMeasuredMm, ...
    focalLengthFresh, ...
    focalLengthDataValid, ...
    cameraModelValid, ...
    focalAtWorkingLowerLimit, ...
    focalAtWorkingUpperLimit, ...
    focalHeadroomMm, ...
    focalFeasible, ...
    validLeft, ...
    validStereoQualified, ...
    ekfPredictionValid, ...
    resetSafe, ...
    focalCommandOutwardAtWorkingLimit, ...
    focalRateUsageGuaranteedCmd, ...
    focalRateUsageHardCmd, ...
    rightReacquireActive, ...
    Ts, ...
    zoomPriorityEnable, ...
    armDepthRampTime, ...
    scaleErrorEnterThreshold, ...
    scaleErrorExitThreshold, ...
    scaleSettledHoldTime, ...
    disturbanceConfirmTime, ...
    zoomOnlyMaxTime)
%#codegen
% V2 Zoom优先级状态机。
% 所有配置参数均由外部 Constant 块输入。
%
% schedulerMode:
% 0 INITIALIZE
% 1 ZOOM_FIRST
% 2 ARM_RECOVERY
% 3 FULL_TRACK
% 4 SAFE_HOLD
% 5 RIGHT_REACQUIRE

persistent mode
persistent zoomTimer
persistent settledTimer
persistent rampTimer
persistent reason
persistent disturbanceTimer
persistent validLast
persistent rateTimer

if isempty(mode)
    mode = 0;
    zoomTimer = 0;
    settledTimer = 0;
    rampTimer = 0;
    reason = 0;
    disturbanceTimer = 0;
    validLast = 0;
    rateTimer = 0;
end

if resetSafe > 0.5
    mode = 0;
    zoomTimer = 0;
    settledTimer = 0;
    rampTimer = 0;
    reason = 0;
    disturbanceTimer = 0;
    validLast = 0;
    rateTimer = 0;
end

depthTaskWeight = 0;
newDisturbanceDetected = 0;

centerValid = ...
    validLeft > 0.5;

focalStateValid = ...
    focalLengthDataValid > 0.5 && ...
    cameraModelValid > 0.5;

depthReady = ...
    validStereoQualified > 0.5 && ...
    ekfPredictionValid > 0.5 && ...
    rightReacquireActive <= 0.5;

maximumScaleError = ...
    max(abs(scaleError));

%% 中心任务无效
if ~centerValid

    mode = 4;
    depthTaskWeight = 0;

    zoomTimer = 0;
    settledTimer = 0;
    rampTimer = 0;
    disturbanceTimer = 0;
    rateTimer = 0;
    validLast = 0;

%% 焦距数据或相机模型无效
elseif ~focalStateValid

    mode = 4;
    depthTaskWeight = 0;

    zoomTimer = 0;
    settledTimer = 0;
    rampTimer = 0;
    disturbanceTimer = 0;
    rateTimer = 0;
    validLast = 0;

%% 双目深度暂不可用
elseif ~depthReady

    mode = 5;
    depthTaskWeight = 0;

    zoomTimer = 0;
    settledTimer = 0;
    rampTimer = 0;
    disturbanceTimer = 0;
    rateTimer = 0;
    validLast = 0;

%% 焦距仅不新鲜：Zoom暂停，深度继续
elseif focalLengthFresh <= 0.5

    mode = 3;
    depthTaskWeight = 1;

    zoomTimer = 0;
    settledTimer = 0;
    rampTimer = armDepthRampTime;
    disturbanceTimer = 0;
    rateTimer = 0;
    reason = 0;
    validLast = 1;

%% 禁用Zoom优先级
elseif zoomPriorityEnable <= 0.5

    mode = 3;
    depthTaskWeight = 1;

    zoomTimer = 0;
    settledTimer = 0;
    rampTimer = armDepthRampTime;
    disturbanceTimer = 0;
    rateTimer = 0;
    reason = 0;
    validLast = 1;

else

    if validLast < 0.5 && ...
            (mode == 4 || mode == 5)

        mode = 1;

        zoomTimer = 0;
        settledTimer = 0;
        rampTimer = 0;
        disturbanceTimer = 0;
        rateTimer = 0;
        reason = 0;
    end

    if mode == 0

        if maximumScaleError > ...
                scaleErrorEnterThreshold

            mode = 1;
            depthTaskWeight = 0;

        else
            mode = 3;
            depthTaskWeight = 1;
        end

    elseif mode == 1

        depthTaskWeight = 0;
        zoomTimer = zoomTimer + Ts;

        if maximumScaleError <= ...
                scaleErrorExitThreshold

            settledTimer = ...
                settledTimer + Ts;
        else
            settledTimer = 0;
        end

        if any( ...
                focalRateUsageGuaranteedCmd >= 1)

            rateTimer = ...
                rateTimer + Ts;
        else
            rateTimer = 0;
        end

        if any(focalRateUsageHardCmd >= 1)

            mode = 2;
            reason = 6;
            rampTimer = 0;
            rateTimer = 0;

        elseif rateTimer >= ...
                disturbanceConfirmTime && ...
                maximumScaleError > ...
                scaleErrorExitThreshold

            mode = 2;
            reason = 5;
            rampTimer = 0;
            rateTimer = 0;

        elseif settledTimer >= ...
                scaleSettledHoldTime

            mode = 2;
            reason = 1;
            rampTimer = 0;
            rateTimer = 0;

        elseif any( ...
                focalCommandOutwardAtWorkingLimit > 0.5)

            mode = 2;
            reason = 7;
            rampTimer = 0;
            rateTimer = 0;

        elseif zoomTimer >= ...
                disturbanceConfirmTime && ...
                any(focalFeasible < 0.5)

            mode = 2;
            reason = 3;
            rampTimer = 0;
            rateTimer = 0;

        elseif zoomTimer >= zoomOnlyMaxTime

            mode = 2;
            reason = 4;
            rampTimer = 0;
            rateTimer = 0;
        end

    elseif mode == 2

        rampTimer = min( ...
            rampTimer + Ts, ...
            armDepthRampTime);

        rampFraction = min(max( ...
            rampTimer / max( ...
                armDepthRampTime, ...
                Ts), ...
            0), 1);

        depthTaskWeight = ...
            rampFraction * ...
            rampFraction * ...
            (3 - 2*rampFraction);

        if depthTaskWeight >= 1 - 1e-6
            mode = 3;
            depthTaskWeight = 1;
            disturbanceTimer = 0;
        end

    elseif mode == 3

        depthTaskWeight = 1;

        if maximumScaleError >= ...
                scaleErrorEnterThreshold

            depthTaskWeight = 0;

            disturbanceTimer = ...
                disturbanceTimer + Ts;
        else
            disturbanceTimer = 0;
        end

        if disturbanceTimer >= ...
                disturbanceConfirmTime

            mode = 1;
            depthTaskWeight = 0;

            zoomTimer = 0;
            settledTimer = 0;
            rampTimer = 0;
            disturbanceTimer = 0;
            rateTimer = 0;
            reason = 0;

            newDisturbanceDetected = 1;
        end

    else

        mode = 1;
        depthTaskWeight = 0;

        zoomTimer = 0;
        settledTimer = 0;
        rampTimer = 0;
        disturbanceTimer = 0;
        rateTimer = 0;
        reason = 0;
    end

    validLast = 1;
end

schedulerMode = mode;

zoomPriorityActive = ...
    double(mode == 1);

zoomPriorityTimer = ...
    zoomTimer;

scaleSettledTimer = ...
    settledTimer;

armRecoveryReason = ...
    reason;

%% 有限值保护
diagnosticFinite = all(isfinite([
    depthTaskWeight
    schedulerMode
    zoomPriorityTimer
    scaleSettledTimer
    depthErrorDelayed
    focalLengthMeasuredMm
    focalHeadroomMm
    focalAtWorkingLowerLimit
    focalAtWorkingUpperLimit
    focalLengthFresh
    focalLengthDataValid
    cameraModelValid
    Ts
    zoomPriorityEnable
    armDepthRampTime
    scaleErrorEnterThreshold
    scaleErrorExitThreshold
    scaleSettledHoldTime
    disturbanceConfirmTime
    zoomOnlyMaxTime
]));

if ~diagnosticFinite

    mode = 4;
    zoomTimer = 0;
    settledTimer = 0;
    rampTimer = 0;
    reason = 0;
    disturbanceTimer = 0;
    validLast = 0;
    rateTimer = 0;

    depthTaskWeight = 0;
    schedulerMode = 4;
    zoomPriorityActive = 0;
    zoomPriorityTimer = 0;
    scaleSettledTimer = 0;
    armRecoveryReason = 0;
    newDisturbanceDetected = 0;
end
end
